simulink model "task1"  (R2024a)
settings: Solver=VariableStepAuto  StartTime=0.0  StopTime=10  RelTol=1e-3
undefined symbols (not defined in the file): K_CO, K_FB, T
settings Model: Creator=vladislav  LastModifiedBy=vladislav

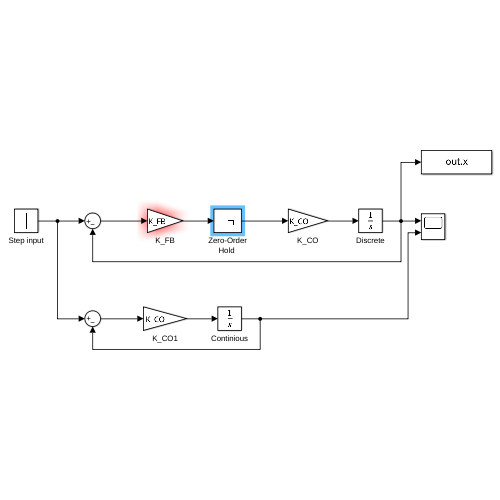
[thumbnail: Simulink's stored preview of the top-level diagram]
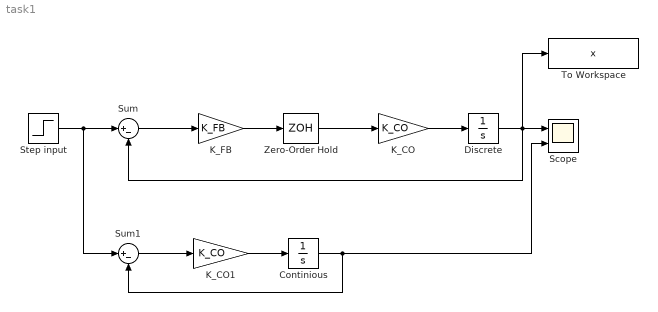
== system task1 ==
  Continious : Integrator
  Discrete : Integrator
  K_CO : Gain  Gain=K_CO
  K_CO1 : Gain  Gain=K_CO
  K_FB : Gain  Gain=K_FB
  Scope : Scope  NumInputPorts=2
  Step input : Step  Before=1  SampleTime=0.0001
  Sum : Sum  Inputs=|+-
  Sum1 : Sum  Inputs=|+-
  To Workspace : ToWorkspace  VariableName=x  SaveFormat=Timeseries  SampleTime=-1
  "Zero-Order Hold " : ZeroOrderHold  SampleTime=T
  wires:
  Step input/1 -> Sum1/1, Sum/1
  Sum/1 -> K_FB/1
  K_FB/1 -> "Zero-Order Hold "/1
  "Zero-Order Hold "/1 -> K_CO/1
  K_CO/1 -> Discrete/1
  Sum1/1 -> K_CO1/1
  Continious/1 -> Scope/2, Sum1/2
  K_CO1/1 -> Continious/1
  Discrete/1 -> Sum/2, To Workspace/1, Scope/1
